simulink model "LAB04_B"  (R2023b)
settings: Solver=VariableStepAuto  StartTime=0.0  StopTime=0.02  RelTol=1e-3
undefined symbols (not defined in the file or in its folder): Angle, Magnitude
libraries: spsPowerPhasorLib x4, spsVoltageMeasurementLib x4, spsCurrentMeasurementLib x3, spsLinearTransformerLib x2, spsSeriesRLCBranchLib x2, spsACVoltageSourceLib x1, sps_lib x1
settings Model: Creator=sagar  LastModifiedBy=sagar

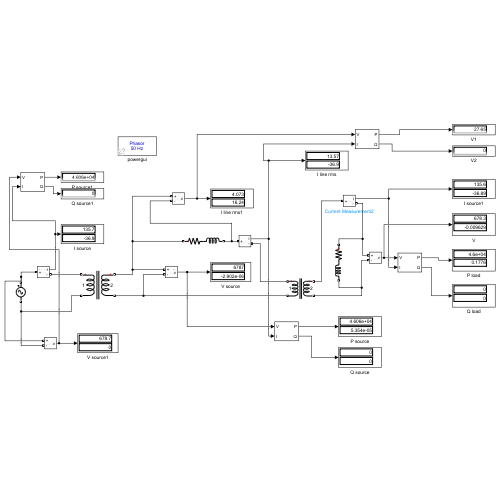
[thumbnail: Simulink's stored preview of the top-level diagram]
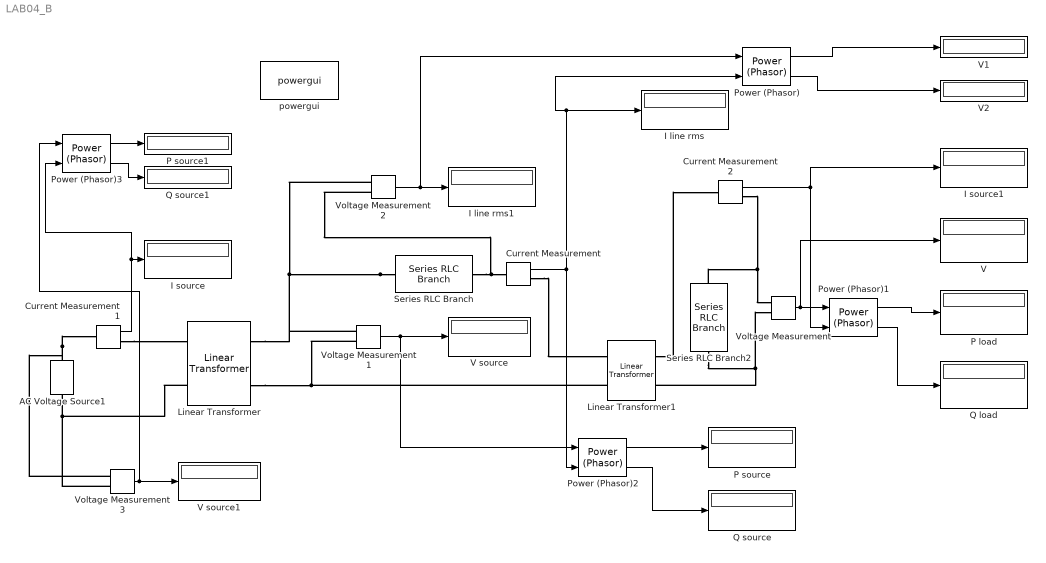
== system LAB04_B ==
  AC Voltage Source1 : spsACVoltageSourceLib/AC Voltage Source  Amplitude=480*1.414  Phase=0  Frequency=50  SampleTime=0  Measurements=None  BusType=swing  Pref=10e3  Qref=0  Qmin=-inf  Qmax=+inf
  Current Measurement : spsCurrentMeasurementLib/Current Measurement  PhasorSimulation=on  OutputType=Magnitude-Angle  PSBequivalent=0
  Current Measurement1 : spsCurrentMeasurementLib/Current Measurement  PhasorSimulation=on  OutputType=Magnitude-Angle  PSBequivalent=0
  Current Measurement2 : spsCurrentMeasurementLib/Current Measurement  PhasorSimulation=on  OutputType=Magnitude-Angle  PSBequivalent=0
  I line rms : Display
  I line rms1 : Display
  I source : Display
  I source1 : Display
  Linear Transformer : spsLinearTransformerLib/Linear Transformer  UNITS=SI  NominalPower=[ 250e6 50 ]  winding1=[480 0.000000001 0.000000001]  winding2=[4800 0.000000001 0.000000001]  ThreeWindings=off  winding3=[3.15e+05 0.7938 0.084225]  RmLm=[1.0804e+06 2866]  Measurements=None  DataType=on
  Linear Transformer1 : spsLinearTransformerLib/Linear Transformer  UNITS=SI  NominalPower=[ 250e6 50 ]  winding1=[4800 0.000000001 0.000000001]  winding2=[480 0.000000001 0.000000001]  ThreeWindings=off  winding3=[3.15e+05 0.7938 0.084225]  RmLm=[1.0804e+06 2866]  Measurements=None  DataType=on
  P load : Display
  P source : Display
  P source1 : Display
  Power (Phasor){,1..3} (4 alike) : spsPowerPhasorLib/Power (Phasor)
      settings: LibrarySourceBlock=|
      | sps_lib/Sensors and Measurements/Power
      | (Phasor)
  Q load : Display
  Q source : Display
  Q source1 : Display
  Series RLC Branch : spsSeriesRLCBranchLib/Series RLC Branch  LConnTagsString=__new0  RConnTagsString=__new0  BranchType=RL  Resistance=0.18  Inductance=0.24/314  SetiL0=off  InitialCurrent=0  Capacitance=0  Setx0=off  InitialVoltage=0  Measurements=None
  Series RLC Branch2 : spsSeriesRLCBranchLib/Series RLC Branch  LConnTagsString=__new0  RConnTagsString=__new0  BranchType=RL  Resistance=4  Inductance=3/314  SetiL0=off  InitialCurrent=0  Capacitance=0  Setx0=off  InitialVoltage=0  Measurements=None
  V : Display
  V source : Display
  V source1 : Display
  V1 : Display
  V2 : Display
  Voltage Measurement{,1..3} (4 alike) : spsVoltageMeasurementLib/Voltage Measurement  PhasorSimulation=on  OutputType=Magnitude-Angle  PSBequivalent=0
  powergui : sps_lib/powergui  Priority=1  SimulationMode=Phasor  SampleTime=50e-6  frequency=50  Iterations=50  frequencyindice=50  Pbase=100e6  ErrMax=1e-4  UnitsV=kV  UnitsW=MW  buscounter=0  FunctionMessages=off  echomessages=off  EnableUseOfTLC=off  CurrentSourceSwitches=off  DisableSnubberDevices=off  DisableRonSwitches=off  DisableVfSwitches=off  DisplayEquations=off  AutomaticDiscreteSolvers=off  SolverType=Tustin/Backward Euler (TBE)  Interpol=off  ExternalGateDelay=off  methode=off  Ts=100  x0status=blocks  SPID=on  SwTol=0  HookPort=off  NonlinearTolerance=1e-4  nMaxIteration=100  ContinueOnMaxIteration=off  RestoreLinks=warning  ResistiveCurrentMeasurement=off  Frange=[0:2:500]  Ylog=off  Xlog=on  ShowGrid=off  save=off  variable=ZData  structure=0  ZoomFFT=off  StartTime=0.0  cycles=1  DisplayStyle=1  fundamental=60  FreqAxis=off  MaxFrequency=1000  frequencyindicesteady=1  RmsSteady=1  display=off
  wires:
  Power (Phasor)1/2 -> Q load/1
  Power (Phasor)/1 -> V1/1
  Power (Phasor)2/2 -> Q source/1
  Power (Phasor)2/1 -> P source/1
  Power (Phasor)1/1 -> P load/1
  Current Measurement/1 -> Power (Phasor)2/2, Power (Phasor)/2, I line rms/1
  Voltage Measurement1/1 -> Power (Phasor)2/1, V source/1
  Power (Phasor)/2 -> V2/1
  Voltage Measurement/1 -> V/1, Power (Phasor)1/1
  Voltage Measurement2/1 -> I line rms1/1, Power (Phasor)/1
  Current Measurement1/1 -> Power (Phasor)3/2, I source/1
  Current Measurement2/1 -> I source1/1, Power (Phasor)1/2
  Voltage Measurement3/1 -> Power (Phasor)3/1, V source1/1
  Power (Phasor)3/1 -> P source1/1
  Power (Phasor)3/2 -> Q source1/1
  connections:
  Series RLC Branch/LConn1 -- Linear Transformer/RConn1 -- Voltage Measurement1/LConn1 -- Voltage Measurement2/LConn1
  Voltage Measurement1/LConn2 -- Linear Transformer/RConn2 -- Linear Transformer1/LConn2
  Current Measurement/RConn1 -- Linear Transformer1/LConn1
  Current Measurement/LConn1 -- Series RLC Branch/RConn1 -- Voltage Measurement2/LConn2
  Linear Transformer/LConn2 -- Voltage Measurement3/LConn2 -- AC Voltage Source1/LConn1
  Linear Transformer1/RConn1 -- Current Measurement2/LConn1
  Series RLC Branch2/RConn1 -- Voltage Measurement/LConn2 -- Linear Transformer1/RConn2
  AC Voltage Source1/RConn1 -- Voltage Measurement3/LConn1 -- Current Measurement1/LConn1
  Current Measurement1/RConn1 -- Linear Transformer/LConn1
  Current Measurement2/RConn1 -- Series RLC Branch2/LConn1 -- Voltage Measurement/LConn1
